simulink model "sample_model"  (R2023a)
settings: Solver=ode5  StartTime=0.0  StopTime=Inf  FixedStep=0.0001  RelTol=1e-3
PostLoadFcn:
  | , if any(exist('dsrtsu_mdlpostloadfcn', 'file') ~= 0), dsrtsu_mdlpostloadfcn('Execute', bdroot); end,
InitFcn:
  | , if any(exist('rtifpga_mdlclblib', 'file') ~= 0), rtifpga_mdlclblib('Init', bdroot); end,
values from neighbouring files (symbols this model uses):
  alpha = 0    [freq_sweep.m]    (also in single_test.m)
  k_harmonics = 7    [freq_sweep.m]    (also in single_test.m)
libraries: rti1202lib_adc_class1 x3, rti1202lib_dac_class1 x2, simulink x2, rti1202lib_base x1
(part 2 of 2)

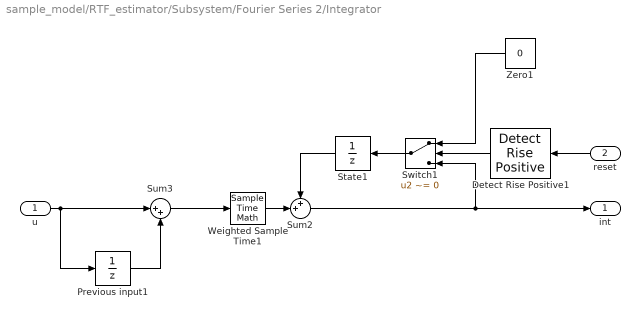
== system sample_model/RTF_estimator/Subsystem/Fourier Series 2/Integrator ==
  u : Inport
  reset : Inport  Port=2
  Detect Rise Positive1 : simulink/Logic and Bit Operations/Detect Rise Positive  vinit=0  OutDataTypeStr=uint8
  Previous input1 : UnitDelay  SampleTime=-1  HasFrameUpgradeWarning=on
  State1 : UnitDelay  SampleTime=-1  HasFrameUpgradeWarning=on
  Sum2 : Sum  Inputs=++|
  Sum3 : Sum  Inputs=|++
  Switch1 : Switch  Criteria=u2 ~= 0  SaturateOnIntegerOverflow=off  InputSameDT=off
  Weighted Sample Time1 : SampleTimeMath  TsampMathOp=*  weightValue=0.5
  Zero1 : Constant  Value=0
  int : Outport
  wires:
  State1/1 -> Sum2/1
  Sum2/1 -> Switch1/3, int/1
  Weighted Sample Time1/1 -> Sum2/2
  Sum3/1 -> Weighted Sample Time1/1
  u/1 -> Sum3/1, Previous input1/1
  Previous input1/1 -> Sum3/2
  reset/1 -> Detect Rise Positive1/1
  Switch1/1 -> State1/1
  Zero1/1 -> Switch1/1
  Detect Rise Positive1/1 -> Switch1/2

== system sample_model/RTF_estimator/Subsystem/Fourier Series 2/Latched first order hold ==
  In : Inport  LatchByDelayingOutsideSignal=on
  Trigger : TriggerPort  VariantControl=(inherit)
  Out : Outport
  wires:
  In/1 -> Out/1

== system sample_model/RTF_estimator1/Subsystem/Fourier Series 2/First order hold ==
  In : Inport  LatchByDelayingOutsideSignal=on
  Trigger : TriggerPort  VariantControl=(inherit)
  Out : Outport
  wires:
  In/1 -> Out/1

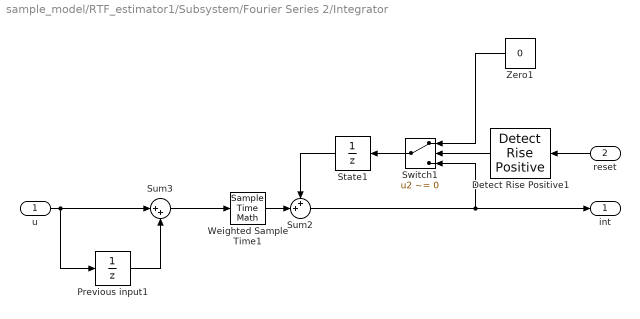
== system sample_model/RTF_estimator1/Subsystem/Fourier Series 2/Integrator ==
  u : Inport
  reset : Inport  Port=2
  Detect Rise Positive1 : simulink/Logic and Bit Operations/Detect Rise Positive  vinit=0  OutDataTypeStr=uint8
  Previous input1 : UnitDelay  SampleTime=-1  HasFrameUpgradeWarning=on
  State1 : UnitDelay  SampleTime=-1  HasFrameUpgradeWarning=on
  Sum2 : Sum  Inputs=++|
  Sum3 : Sum  Inputs=|++
  Switch1 : Switch  Criteria=u2 ~= 0  SaturateOnIntegerOverflow=off  InputSameDT=off
  Weighted Sample Time1 : SampleTimeMath  TsampMathOp=*  weightValue=0.5
  Zero1 : Constant  Value=0
  int : Outport
  wires:
  Detect Rise Positive1/1 -> Switch1/2
  Zero1/1 -> Switch1/1
  Switch1/1 -> State1/1
  reset/1 -> Detect Rise Positive1/1
  Previous input1/1 -> Sum3/2
  u/1 -> Previous input1/1, Sum3/1
  Sum3/1 -> Weighted Sample Time1/1
  Weighted Sample Time1/1 -> Sum2/2
  Sum2/1 -> int/1, Switch1/3
  State1/1 -> Sum2/1

== system sample_model/RTF_estimator1/Subsystem/Fourier Series 2/Latched first order hold ==
  In : Inport  LatchByDelayingOutsideSignal=on
  Trigger : TriggerPort  VariantControl=(inherit)
  Out : Outport
  wires:
  In/1 -> Out/1

== system sample_model/RTI Data/RTI Data Store/RTI Data Store/RTI Data Store ==
  RTI Data Store : Subsystem  mask(RTI_DATA_STORE){}
      mask help:
      | RTI Data Store Block. This block is used by RTI to store internal model dependent data. Deleting this block will result in data loss.
      |
      | NEVER DELETE, COPY, OR MODIFY THIS BLOCK!
      mask Help:
      | RTI Data Store Block. This block is used by RTI to store internal model dependent data. Deleting this block will result in data loss.
      | 
      | NEVER DELETE, COPY, OR MODIFY THIS BLOCK!
      mask Display: text(0.5, 0.5, ' ', 'HorizontalAlignment', 'center');

== system sample_model/RTI Data/RTI Data Store/RTI Data Store/RTI Data Store/RTI Data Store ==

== matlab function sample_model/RTF_estimator/MATLAB Function1 ==
  data: Coeffs input; avgCoeffs output; varCoeffs output
function [avgCoeffs, varCoeffs] = exponentialAverageWithVariance(Coeffs)
% Exponential Moving Average (EMA) and Variance (EMV) for Fourier Coefficients

% Tuning parameter
alpha = 5e-4;  % 0.001 (slow, smooth) to 0.1 (fast, responsive)

% Persistent storage
persistent avg sqAvg
if isempty(avg)
    avg = Coeffs;
    sqAvg = Coeffs.^2;
end

% EMA update
avg = alpha * Coeffs + (1 - alpha) * avg;

% EMA of square
sqAvg = alpha * (Coeffs.^2) + (1 - alpha) * sqAvg;

% Variance = E[x^2] - (E[x])^2
varCoeffs = sqAvg - avg.^2;

% Output
avgCoeffs = avg;
end

== matlab function sample_model/RTF_estimator1/MATLAB Function1 ==
  data: Coeffs input; avgCoeffs output; varCoeffs output
function [avgCoeffs, varCoeffs] = exponentialAverageWithVariance(Coeffs)
% Exponential Moving Average (EMA) and Variance (EMV) for Fourier Coefficients

% Tuning parameter
alpha = 5e-4;  % 0.001 (slow, smooth) to 0.1 (fast, responsive)

% Persistent storage
persistent avg sqAvg
if isempty(avg)
    avg = Coeffs;
    sqAvg = Coeffs.^2;
end

% EMA update
avg = alpha * Coeffs + (1 - alpha) * avg;

% EMA of square
sqAvg = alpha * (Coeffs.^2) + (1 - alpha) * sqAvg;

% Variance = E[x^2] - (E[x])^2
varCoeffs = sqAvg - avg.^2;

% Output
avgCoeffs = avg;
end
